simulink model "test_atan2"  (Simulink 7.6)
settings: Solver=ode45  StartTime=0.0  StopTime=100.0  RelTol=1e-3
libraries: simulink x12
settings Model: Creator=jporter  LastModifiedBy=jporter

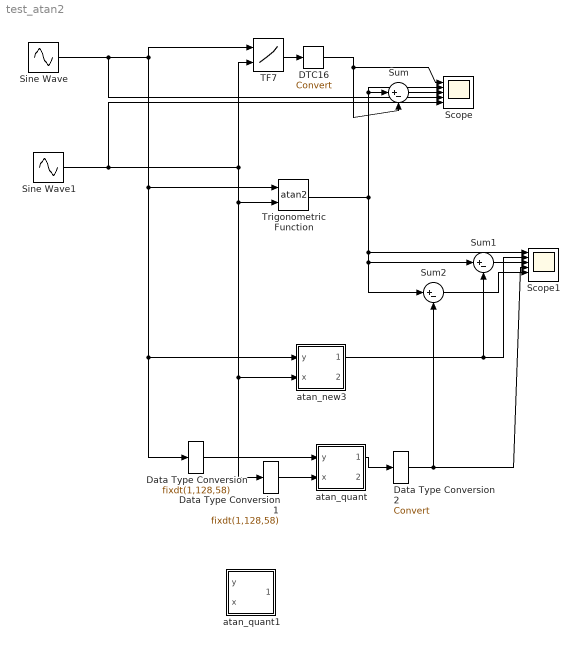
== system test_atan2 ==
  DTC16 : DataTypeConversion
  Data Type Conversion : DataTypeConversion  OutDataTypeStr=fixdt(1,128,58)
  Data Type Conversion1 : DataTypeConversion  OutDataTypeStr=fixdt(1,128,58)
  Data Type Conversion2 : DataTypeConversion
  Scope : Scope  NumInputPorts=5
      settings: YMin=-5~-5~-5~-5~-5  YMax=5~5~5~5~5
  Scope1 : Scope  NumInputPorts=6
      settings: YMin=-5~-5~-5~-5~-5~-5  YMax=5~5~5~5~5~5
  Sine Wave : Sin  Amplitude=2  Frequency=2  SampleTime=0
  Sine Wave1 : Sin  Amplitude=2  Frequency=5  SampleTime=0
  Sum : Sum  Inputs=|+-
  Sum1 : Sum  Inputs=|+-
  Sum2 : Sum  Inputs=|+-
  TF7 : Lookup2D  RowIndex=[ -1000 -10 -sqrt(10) -1 -sqrt(.1) -0.01 0 0.01 sqrt(.1) 1 sqrt(10) 10 1000 ]  ColumnIndex=[ -1000 -10 -sqrt(10) -1 -sqrt(.1) -0.01 0 0.01 sqrt(.1) 1 sqrt(10) 10 1000 ]  Table=[-2.35619449019234 -1.58079599348156 -1.5739585939142 -1.57179632646156 -1.57111255455037 -1.5708063267949 -1.5707963267949 -1.5707863267949 -1.57048009903942 -1.56979632712823 -1.56763405967559 -1.56079666010823 -0.785398163397448;-3.13159298690313 -2.35619449019234 -1.87707369596457 -1.67046497928606 -1.60240856879109 -1.57179632646156 -1.5707963267949 -1.56979632712823 -1.53918408479871 -1.47112767430373 -1.26451895762523 -0.785398163397448 -0.00999966668666524;-3.13843038647049 -2.83531528442012 -2.35619449019234 -1.87707369596457 -1.67046497928606 -1.5739585939142 -1.5707963267949 -1.56763405967559 -1.47112767430373 -1.26451895762523 -0.785398163397448 -0.306277369169669 -0.00316226711930609;-3.14059265392313 -3.04192400109863 -2.83531528442012 -2.35619449019234 -1.87707369596457 -1.58079599348156 -1.5707963267949 -1.56079666010823 -1.26451895762523 -0.785398163397448 -0.306277369169669 -0.099668652491162 -0.000999999666666867;-3.14127642583432 -3.1099804115936 -3.04192400109863 -2.83531528442012 -2.35619449019234 -1.60240856879109 -1.5707963267949 -1.53918408479871 -0.785398163397448 -0.306277369169669 -0.099668652491162 -0.0316122419961912 -0.000316227755475913;-3.14158265358979 -3.14059265392313 -3.13843038647049 -3.13159298690313 -3.1099804115936 -2.35619449019234 -1.5707963267949 -0.785398163397448 -0.0316122419961912 -0.00999966668666524 -0.00316226711930609 -0.000999999666666867 -9.99999999966667e-006;3.14159265358979 3.14159265358979 3.14159265358979 3.14159265358979 3.14159265358979 3.14159265358979 0 0 0 0 0 0 0;3.14158265358979 3.14059265392313 3.13843038647049 3.13159298690313 3.1099804115936 2.35619449019234 1.5707963267949 0.785398163397448 0.0316122419961912 0.00999966668666524 0.00316226711930609 0.000999999666666867 9.99999999966667e-006;3.14127642583432 3.1099804115936 3.04192400109863 2.83531528442012 2.35619449019234 1.60240856879109 1.5707963267949 1.53918408479871 0.785398163397448 0.306277369169669 0.099668652491162 0.0316122419961912 0.000316227755475913;3.14059265392313 3.04192400109863 2.83531528442012 2.35619449019234 1.87707369596457 1.58079599348156 1.5707963267949 1.56079666010823 1.26451895762523 0.785398163397448 0.306277369169669 0.099668652491162 0.000999999666666867;3.13843038647049 2.83531528442012 2.35619449019234 1.87707369596457 1.67046497928606 1.5739585939142 1.5707963267949 1.56763405967559 1.47112767430373 1.26451895762523 0.785398163397448 0.306277369169669 0.00316226711930609;3.13159298690313 2.35619449019234 1.87707369596457 1.67046497928606 1.60240856879109 1.57179632646156 1.5707963267949 1.56979632712823 1.53918408479871 1.47112767430373 1.26451895762523 0.785398163397448 0.00999966668666524;2.35619449019234 1.58079599348156 1.5739585939142 1.57179632646156 1.57111255455037 1.5708063267949 1.5707963267949 1.5707863267949 1.57048009903942 1.56979632712823 1.56763405967559 1.56079666010823 0.785398163397448]
  Trigonometric Function : Trigonometry  Operator=atan2
  atan_new3 : Subsystem
  atan_quant : Subsystem
  atan_quant1 : Subsystem
  wires:
  TF7/1 -> DTC16/1
  Sine Wave/1 -> TF7/1, Trigonometric Function/1, Data Type Conversion/1, atan_new3/1(y), Scope/4
  Sine Wave1/1 -> TF7/2, Trigonometric Function/2, Data Type Conversion1/1, atan_new3/2(x), Scope/5
  DTC16/1 -> Scope/1, Sum/2
  Trigonometric Function/1 -> Scope/2, Sum/1, Scope1/1, Sum1/1, Sum2/1
  Sum/1 -> Scope/3
  Sum1/1 -> Scope1/3
  atan_new3/1(atan2) -> Sum1/2, Scope1/2
  atan_quant/1(atan2) -> Data Type Conversion2/1
  Sum2/1 -> Scope1/5
  Data Type Conversion/1 -> atan_quant/1(y)
  Data Type Conversion1/1 -> atan_quant/2(x)
  Data Type Conversion2/1 -> Scope1/4, Sum2/2

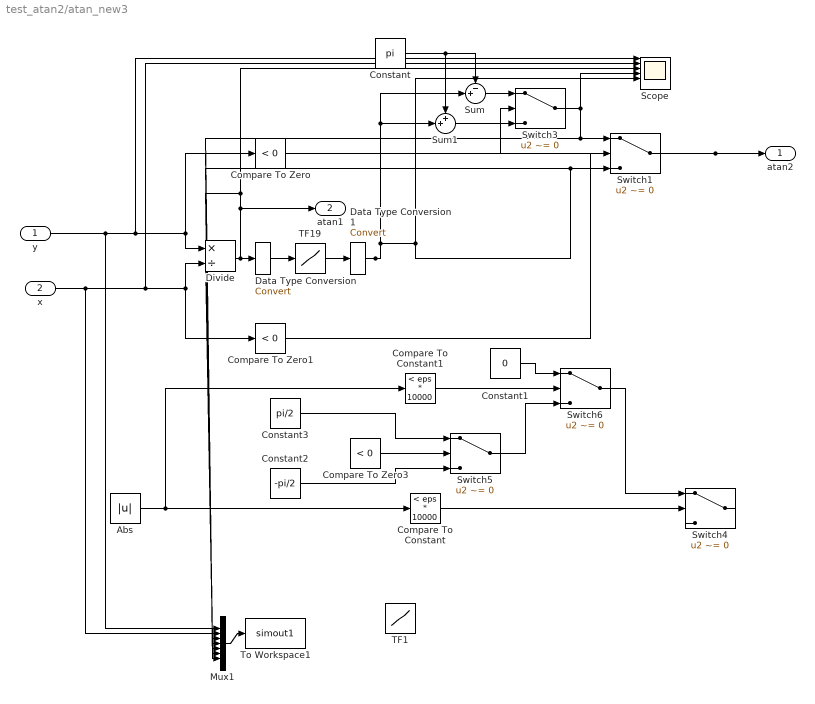
== system test_atan2/atan_new3 ==
  y : Inport
  x : Inport  Port=2
  Abs : Abs
  Compare To Constant : simulink/Logic and Bit Operations/Compare To Constant  SystemSampleTime=-1  relop=<  const=eps * 10000  LogicOutDataTypeMode=uint8
  Compare To Constant1 : simulink/Logic and Bit Operations/Compare To Constant  SystemSampleTime=-1  relop=<  const=eps * 10000  LogicOutDataTypeMode=uint8
  Compare To Zero : simulink/Logic and Bit Operations/Compare To Zero  SystemSampleTime=-1  relop=<  LogicOutDataTypeMode=uint8
  Compare To Zero1 : simulink/Logic and Bit Operations/Compare To Zero  SystemSampleTime=-1  relop=<  LogicOutDataTypeMode=uint8
  Compare To Zero3 : simulink/Logic and Bit Operations/Compare To Zero  SystemSampleTime=-1  relop=<  LogicOutDataTypeMode=uint8
  Constant : Constant  Value=pi  OutDataTypeStr=double
  Constant1 : Constant  Value=0  OutDataTypeStr=double
  Constant2 : Constant  Value=-pi/2  OutDataTypeStr=double
  Constant3 : Constant  Value=pi/2  OutDataTypeStr=double
  Data Type Conversion : DataTypeConversion
  Data Type Conversion1 : DataTypeConversion
  Divide : Product  Inputs=*/  OutDataTypeStr=double
  Mux1 : Mux  Inputs=7
  Scope : Scope  NumInputPorts=7
      settings: YMin=-5~-5~-5~-5~-5~-5~-5  YMax=5~5~5~5~5~5~5  SaveName=ScopeData3
  Sum : Sum  Inputs=-+|  OutDataTypeStr=double
  Sum1 : Sum  Inputs=++|  OutDataTypeStr=double
  Switch{1,3..6} (5 alike) : Switch  Criteria=u2 ~= 0  OutDataTypeStr=double
  TF1 : Lookup  InputValues=[-5:5]  Table=atan([-5:5])  OutDataTypeStr=double
  TF19 : Lookup  InputValues=[-10 -5 -2.5:.1:-.11 -.1:.001:.1 .11:.1:2.5 5 10]  Table=[ -pi/2 atan([-5 -2.5:.1:-.11 -.1:.001:.1 .11:.1:2.5 5]) pi/2 ]  LookUpMeth=Interpolation-Use End Values  OutDataTypeStr=double
  To Workspace1 : ToWorkspace  VariableName=simout1  SampleTime=-1  SaveFormat=Structure
  atan2 : Outport
  atan1 : Outport  Port=2
  wires:
  y/1 -> Divide/1, Compare To Zero/1, Scope/1, Mux1/1
  x/1 -> Divide/2, Compare To Zero1/1, Scope/2, Mux1/2
  Divide/1 -> Data Type Conversion/1, atan1/1, Scope/3, Mux1/3
  Switch3/1 -> Scope/4, Switch1/1, Mux1/5
  Constant/1 -> Sum1/1, Sum/1
  Sum/1 -> Switch3/1
  Sum1/1 -> Switch3/3
  Compare To Zero/1 -> Switch3/2
  Compare To Zero1/1 -> Switch1/2
  Compare To Constant/1 -> Switch4/2
  Compare To Zero3/1 -> Switch5/2
  Compare To Constant1/1 -> Switch6/2
  Switch5/1 -> Switch6/3
  Constant1/1 -> Switch6/1
  Switch6/1 -> Switch4/1
  Constant2/1 -> Switch5/3
  Constant3/1 -> Switch5/1
  Data Type Conversion1/1 -> Sum1/2, Sum/2, Scope/5, Switch1/3, Mux1/6, Mux1/4
  Abs/1 -> Compare To Constant/1, Compare To Constant1/1
  Data Type Conversion/1 -> TF19/1
  TF19/1 -> Data Type Conversion1/1
  Switch1/1 -> atan2/1, Mux1/7
  Mux1/1 -> To Workspace1/1

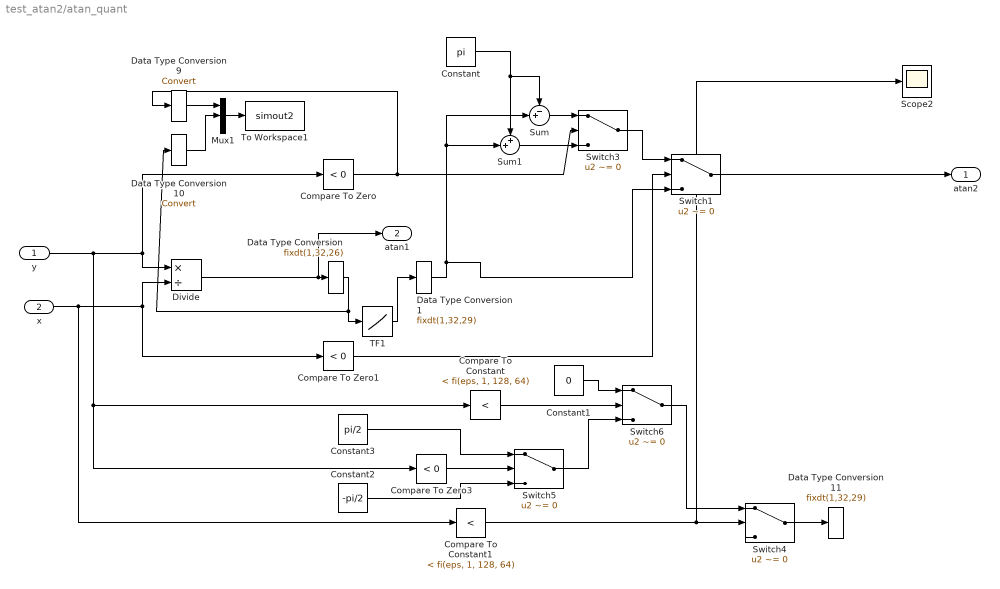
== system test_atan2/atan_quant ==
  y : Inport
  x : Inport  Port=2
  Compare To Constant : simulink/Logic and Bit Operations/Compare To Constant  SystemSampleTime=-1  relop=<  const=fi(eps, 1, 128, 64)  LogicOutDataTypeMode=boolean
  Compare To Constant1 : simulink/Logic and Bit Operations/Compare To Constant  SystemSampleTime=-1  relop=<  const=fi(eps, 1, 128, 64)  LogicOutDataTypeMode=boolean
  Compare To Zero : simulink/Logic and Bit Operations/Compare To Zero  SystemSampleTime=-1  relop=<  LogicOutDataTypeMode=uint8
  Compare To Zero1 : simulink/Logic and Bit Operations/Compare To Zero  SystemSampleTime=-1  relop=<  LogicOutDataTypeMode=uint8
  Compare To Zero3 : simulink/Logic and Bit Operations/Compare To Zero  SystemSampleTime=-1  relop=<  LogicOutDataTypeMode=uint8
  Constant : Constant  Value=pi  OutDataTypeStr=Inherit: Inherit via back propagation
  Constant1 : Constant  Value=0  OutDataTypeStr=Inherit: Inherit via back propagation
  Constant2 : Constant  Value=-pi/2  OutDataTypeStr=Inherit: Inherit via back propagation
  Constant3 : Constant  Value=pi/2  OutDataTypeStr=Inherit: Inherit via back propagation
  Data Type Conversion : DataTypeConversion  OutDataTypeStr=fixdt(1,32,26)  SaturateOnIntegerOverflow=on
  Data Type Conversion1 : DataTypeConversion  OutDataTypeStr=fixdt(1,32,29)
  Data Type Conversion10 : DataTypeConversion
  Data Type Conversion11 : DataTypeConversion  OutDataTypeStr=fixdt(1,32,29)
  Data Type Conversion9 : DataTypeConversion
  Divide : Product  Inputs=*/  SaturateOnIntegerOverflow=on  OutDataTypeStr=Inherit: Same as first input
  Mux1 : Mux  Inputs=3
  Scope2 : Scope
      settings: YMin=-1  YMax=2  SaveName=ScopeData2
  Sum : Sum  Inputs=-+|  OutDataTypeStr=Inherit: Inherit via back propagation
  Sum1 : Sum  Inputs=++|  OutDataTypeStr=Inherit: Inherit via back propagation
  Switch{1,3..6} (5 alike) : Switch  Criteria=u2 ~= 0  OutDataTypeStr=Inherit: Inherit via back propagation
  TF1 : Lookup  InputValues=fi([-10:.8:10], 1, 32, 26)  Table=fi([ -pi/2 atan([-(10-.8):.8:(10-.8)]) pi/2 ], 1, 32, 29)  LookUpMeth=Interpolation-Use End Values  OutDataTypeStr=fixdt(1,32,29)
  To Workspace1 : ToWorkspace  VariableName=simout2  SampleTime=-1  SaveFormat=Structure
  atan2 : Outport
  atan1 : Outport  Port=2
  wires:
  y/1 -> Compare To Zero3/1, Compare To Constant/1, Divide/1, Compare To Zero/1
  x/1 -> Compare To Constant1/1, Divide/2, Compare To Zero1/1
  Divide/1 -> Data Type Conversion/1, atan1/1
  Switch3/1 -> Switch1/1
  TF1/1 -> Data Type Conversion1/1
  Constant/1 -> Sum1/1, Sum/1
  Sum/1 -> Switch3/1
  Sum1/1 -> Switch3/3
  Compare To Zero/1 -> Switch3/2, Data Type Conversion9/1
  Compare To Zero1/1 -> Switch1/2
  Data Type Conversion/1 -> TF1/1, Data Type Conversion10/1
  Data Type Conversion1/1 -> Sum/2, Sum1/2, Switch1/3
  Switch1/1 -> atan2/1
  Mux1/1 -> To Workspace1/1
  Data Type Conversion9/1 -> Mux1/1
  Data Type Conversion10/1 -> Mux1/2
  Compare To Constant1/1 -> Switch4/2, Scope2/1
  Compare To Zero3/1 -> Switch5/2
  Compare To Constant/1 -> Switch6/2
  Switch5/1 -> Switch6/3
  Constant1/1 -> Switch6/1
  Switch6/1 -> Switch4/1
  Constant2/1 -> Switch5/3
  Constant3/1 -> Switch5/1
  Switch4/1 -> Data Type Conversion11/1

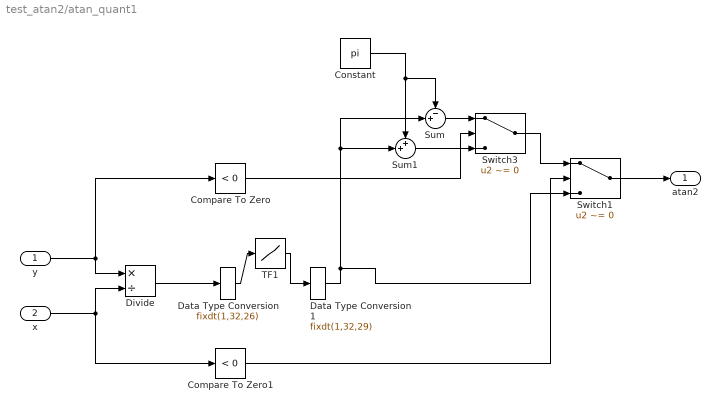
== system test_atan2/atan_quant1 ==
  y : Inport
  x : Inport  Port=2
  Compare To Zero : simulink/Logic and Bit Operations/Compare To Zero  SystemSampleTime=-1  relop=<  LogicOutDataTypeMode=uint8
  Compare To Zero1 : simulink/Logic and Bit Operations/Compare To Zero  SystemSampleTime=-1  relop=<  LogicOutDataTypeMode=uint8
  Constant : Constant  Value=pi  OutDataTypeStr=Inherit: Inherit via back propagation
  Data Type Conversion : DataTypeConversion  OutDataTypeStr=fixdt(1,32,26)  SaturateOnIntegerOverflow=on
  Data Type Conversion1 : DataTypeConversion  OutDataTypeStr=fixdt(1,32,29)
  Divide : Product  Inputs=*/  SaturateOnIntegerOverflow=on  OutDataTypeStr=Inherit: Same as first input
  Sum : Sum  Inputs=-+|  OutDataTypeStr=Inherit: Inherit via back propagation
  Sum1 : Sum  Inputs=++|  OutDataTypeStr=Inherit: Inherit via back propagation
  Switch1 : Switch  Criteria=u2 ~= 0  OutDataTypeStr=Inherit: Inherit via back propagation
  Switch3 : Switch  Criteria=u2 ~= 0  OutDataTypeStr=Inherit: Inherit via back propagation
  TF1 : Lookup  InputValues=fi([-10:.8:10], 1, 32, 26)  Table=fi([ -pi/2 atan([-(10-.8):.8:(10-.8)]) pi/2 ], 1, 32, 29)  LookUpMeth=Interpolation-Use End Values  OutDataTypeStr=fixdt(1,32,29)
  atan2 : Outport
  wires:
  y/1 -> Divide/1, Compare To Zero/1
  x/1 -> Divide/2, Compare To Zero1/1
  Divide/1 -> Data Type Conversion/1
  Switch3/1 -> Switch1/1
  TF1/1 -> Data Type Conversion1/1
  Constant/1 -> Sum1/1, Sum/1
  Sum/1 -> Switch3/1
  Sum1/1 -> Switch3/3
  Compare To Zero/1 -> Switch3/2
  Compare To Zero1/1 -> Switch1/2
  Data Type Conversion/1 -> TF1/1
  Data Type Conversion1/1 -> Sum/2, Sum1/2, Switch1/3
  Switch1/1 -> atan2/1
